simulink subsystem "VCU"  (R2025b)
settings: Solver=VariableStepAuto  StartTime=0.0  StopTime=10.0  RelTol=1e-3
(part 2 of 2)

== stateflow chart VCU/Control_Logic/Torque_Display/Torque_Display ==
  state No_Display
    during:
    if Torque_Display > 0
    Torque_Display = Torque_Display - 1;
    end
  state Yes_Display
    during:
    if Brake == true && Torque_Display > 0
    Torque_Display = Torque_Display - 1;
    elseif Brake == false && Torque_Display < Torque_Command
    Torque_Display = Torque_Display + 1;
    elseif Brake == false && Torque_Display > Torque_Command
    Torque_Display = Torque_Display - 1;
    end
  (default) -> No_Display
  No_Display -> Yes_Display : [uC_State == UC_State.MC_Active]
  Yes_Display -> No_Display : [uC_State ~= UC_State.MC_Active]
  data: uC_State input; Brake input; Torque_Command input; Torque_Display output =0
